simulink model "motor_scoping"  (R2024a)
settings: Solver=VariableStepAuto  StartTime=0.0  StopTime=10.0  RelTol=1e-3
model workspace (MAT data in the model file):
  G = Simulink.Parameter
  G.Value = 1
  G.Complexity = 'real'
  G.Dimensions = [1 1]
  G.DataType = 'auto'
settings Model: Creator=maxhu  LastModifiedBy=maxhu

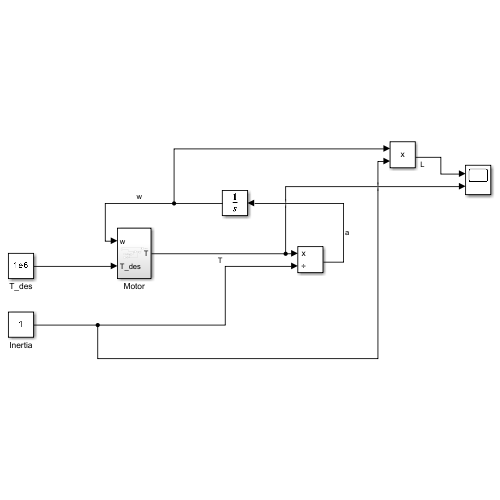
[thumbnail: Simulink's stored preview of the top-level diagram]
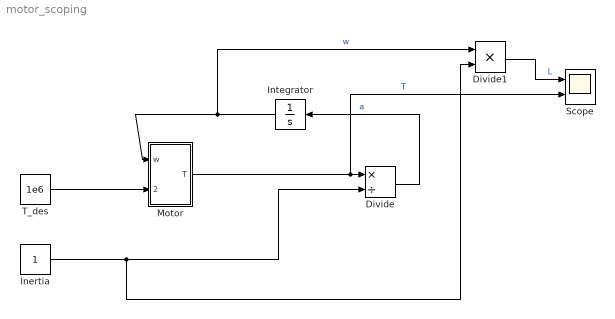
== system motor_scoping ==
  Divide : Product  Inputs=*/
  Divide1 : Product  Inputs=**
  Inertia : Constant
  Integrator : Integrator
  Motor : Subsystem
  Scope : Scope  NumInputPorts=2
  T_des : Constant  Value=1e6
  wires:
  Integrator/1 -> Divide1/1, Motor/1(w)  "w"
  Motor/1(T) -> Scope/2, Divide/1  "T"
  Divide/1 -> Integrator/1  "a"
  Inertia/1 -> Divide1/2, Divide/2
  T_des/1 -> Motor/2(T_des)
  Divide1/1 -> Scope/1  "L"

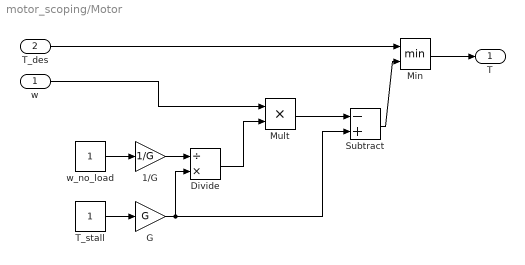
== system motor_scoping/Motor ==
  w : Inport
  T_des : Inport  Port=2
  1/G : Gain  Gain=1/G
  Divide : Product  Inputs=/*
  G : Gain  Gain=G
  Min : MinMax  Inputs=2
  Mult : Product  Inputs=**
  Subtract : Sum  Inputs=-+
  T_stall : Constant
  w_no_load : Constant
  T : Outport
  wires:
  Min/1 -> T/1
  w/1 -> Mult/1
  T_stall/1 -> G/1
  Divide/1 -> Mult/2
  w_no_load/1 -> 1/G/1
  Mult/1 -> Subtract/1
  T_des/1 -> Min/1
  Subtract/1 -> Min/2
  G/1 -> Subtract/2, Divide/2
  1/G/1 -> Divide/1
